simulink model "Control_Block"  (R2022a)
settings: Solver=FixedStepAuto  StartTime=0.0  StopTime=end_time  FixedStep=dt  RelTol=1e-3
values from neighbouring files (symbols this model uses):
  Area = pi() * r0^2    [Main_PD_Control.m]    (also in Test_code.m; main.m = 1.25663706144e-05; main2.m = 1.25663706144e-05)
  Cd = 0.42    [Main_PD_Control.m]    (also in Test_code.m; main.m = 1.05; main2.m = 1.05)
  dt = 0.01    [Main_PD_Control.m]    (also in Test_code.m; load_parameter.m; main.m; main2.m = 0.001)
  K_d = 10    [Main_PD_Control.m]    (also in Test_code.m = 0; main.m; main2.m)
  K_p = 100    [Main_PD_Control.m]    (also in Test_code.m; main.m = 500; main2.m)
  refer_Velo_mag = total_Length / total_Time    (= 0)    [Main_PD_Control.m]    (also in Test_code.m; main.m; main2.m)
  rho = 1000    [Main_PD_Control.m]    (also in Test_code.m; testcode_2d.m = 2700)
settings Model: Creator=zhong  LastModifiedBy=normanzmz
settings DebuggingCC: UnconnectedInputMsg=warning  UnconnectedOutputMsg=warning  UnconnectedLineMsg=warning
settings RTWCC: DLArmComputeVersion=19.05

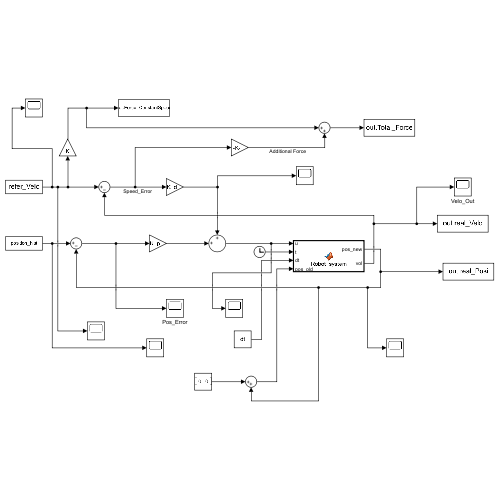
[thumbnail: Simulink's stored preview of the top-level diagram]
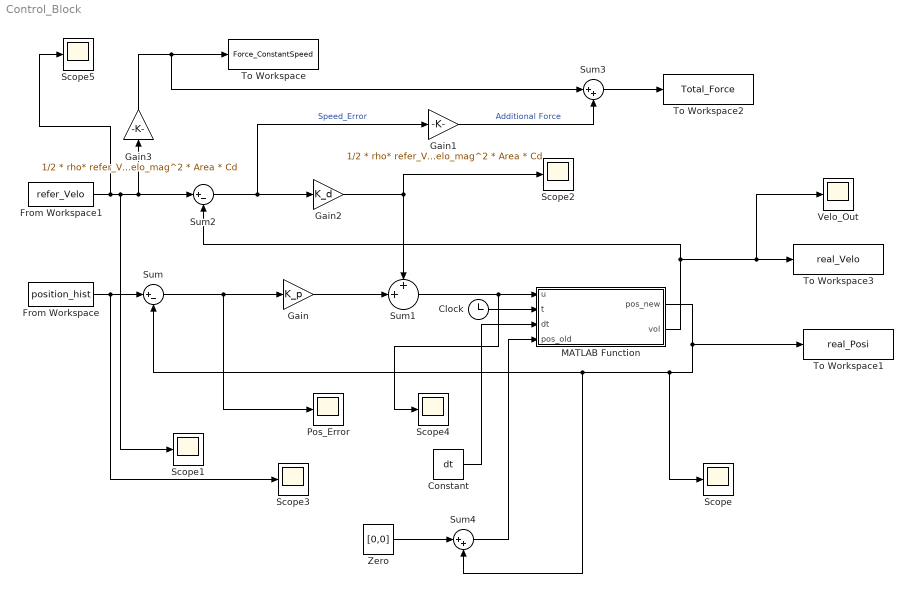
== system Control_Block ==
  Clock : Clock
  Constant : Constant  Value=dt
  From Workspace : FromWorkspace  VariableName=position_hist
  From Workspace1 : FromWorkspace  VariableName=refer_Velo
  Gain : Gain  Gain=K_p
  Gain1 : Gain  Gain=1/2 * rho* refer_Velo_mag^2 * Area * Cd
  Gain2 : Gain  Gain=K_d
  Gain3 : Gain  Gain=1/2 * rho* refer_Velo_mag^2 * Area * Cd
  MATLAB Function : MATLAB Function  TreatAsAtomicUnit=on
  Pos_Error : Scope
  Scope{,1..5} (6 alike) : Scope
  Sum : Sum  Inputs=|+-
  Sum1 : Sum  Inputs=++|
  Sum2 : Sum  Inputs=|+-
  Sum3 : Sum  Inputs=|++
  Sum4 : Sum  Inputs=|++
  To Workspace : ToWorkspace  VariableName=Force_ConstantSpeed  SaveFormat=Timeseries  SampleTime=-1
  To Workspace1 : ToWorkspace  VariableName=real_Posi  SaveFormat=Timeseries  SampleTime=-1
  To Workspace2 : ToWorkspace  VariableName=Total_Force  SaveFormat=Timeseries  SampleTime=-1
  To Workspace3 : ToWorkspace  VariableName=real_Velo  SaveFormat=Timeseries  SampleTime=-1
  Velo_Out : Scope
  Zero : Constant  Value=[0,0]  OutDataTypeStr=Inherit: Inherit via back propagation
  wires:
  From Workspace/1 -> Scope3/1, Sum/1
  Sum/1 -> Pos_Error/1, Gain/1
  Gain/1 -> Sum1/2
  Sum2/1 -> Gain1/1, Gain2/1  "Speed_Error"
  Gain2/1 -> Sum1/1, Scope2/1
  Sum1/1 -> Scope4/1, MATLAB Function/1(u)
  Clock/1 -> MATLAB Function/2(t)
  MATLAB Function/1(pos_new) -> To Workspace1/1, Sum4/2, Sum/2, Scope/1
  MATLAB Function/2(vol) -> Velo_Out/1, To Workspace3/1, Sum2/2
  From Workspace1/1 -> Scope5/1, Scope1/1, Sum2/1, Gain3/1
  Gain3/1 -> Sum3/1, To Workspace/1
  Gain1/1 -> Sum3/2  "Additional Force"
  Sum3/1 -> To Workspace2/1
  Constant/1 -> MATLAB Function/3(dt)
  Zero/1 -> Sum4/1
  Sum4/1 -> MATLAB Function/4(pos_old)

== matlab function Control_Block/MATLAB Function ==
  data: u input; pos_new output; vol output; t input; dt input; pos_old input
function [pos_new,vol] = Robot_system(u,t,dt,pos_old)


disturbance = sin(10*t) * 0;

pos_new = u + disturbance

vol = (pos_new -pos_old)/dt;
